simulink model "latest_coil"  (R2021b)
settings: Solver=FixedStepAuto  StartTime=-8e-3  StopTime=8e-3  FixedStep=1e-4  RelTol=1e-3
undefined symbols (not defined in the file or in its folder): X, Y, Z
libraries: sm_lib x15, nesl_utility x1
(part 2 of 2)

== matlab function latest_coil/Outer Coil/Coil 1/MATLAB Function3 ==
  data: X input; Hx_yp output; Y input; Z input; I input; Hy_yp output; Hz_yp output; Hx_yn output; Hy_yn output; Hz_yn output
function [Hx_yp, Hy_yp, Hz_yp, Hx_yn, Hy_yn, Hz_yn] = field_y(X, Y, Z, I)
n = 1;
gy = 520e-6;
% gx = 675e-6;
gz = 0;
m0 = 4*pi*1e-7;
k = 0.4e-3;
yp1 = -0.6e-3 - (n-1)*k;
yp2 = 0.6e-3 - (n-1)*k;
a_xp = gy;
a_zp = gz;
k_yp = 1./(4*pi*((a_xp-X).^2+(a_zp-Z).^2));
kyp = (yp2-Y)./((yp2-Y).^2+(a_xp-X).^2+(a_zp-Z).^2).^0.5;
k_2yp = (yp1-Y)./((yp1-Y).^2+(a_xp-X).^2+(a_zp-Z).^2).^0.5;

Hx_yp = -((a_zp-Z).*k_yp.*(kyp - k_2yp))*I*m0;
Hy_yp = zeros(size(X,1),size(Y,1),size(Z,1));
Hz_yp = (-(a_xp-X).*k_yp.*(kyp - k_2yp))*I*m0;

a_xn = -gy;
yn1 = -0.8e-3 - (n-1)*k;
yn2 = 0.8e-3 - (n-1)*k;
k_yn = 1./(4*pi*((a_xn-X).^2+(a_zp-Z).^2));
kyn = (yn2-Y)./((yn2-Y).^2+(a_xn-X).^2+(a_zp-Z).^2).^0.5;
k_2yn = (yn1-Y)./((yn1-Y).^2+(a_xn-X).^2+(a_zp-Z).^2).^0.5;

Hx_yn = ((a_zp-Z).*k_yn.*(kyn - k_2yn))*I*m0;
Hy_yn = zeros(size(X,1),size(Y,1),size(Z,1));
Hz_yn = ((a_xn-X).*k_yn.*(kyn - k_2yn))*I*m0;

end

== matlab function latest_coil/Outer Coil/Coil 1/MATLAB Function4 ==
  data: Hx_xp input; Hy_xp input; Hz_xp input; Hx output; Hx_xn input; Hy_xn input; Hy output; Hz output; Hz_xn input; Hx_yp input; Hy_yp input; Hz_yp input; Hx_yn input; Hy_yn input; Hz_yn input
function [Hx, Hy, Hz] = field_sum(Hx_xp, Hy_xp, Hz_xp, Hx_xn, Hy_xn, Hz_xn, Hx_yp, Hy_yp, Hz_yp, Hx_yn, Hy_yn, Hz_yn)
Hx = Hx_xp + Hx_xn + Hx_yp + Hx_yn;
Hy = Hy_xp + Hy_xn + Hy_yp + Hy_yn;
Hz = Hz_xp + Hz_xn + Hz_yp + Hz_yn;
end

== matlab function latest_coil/Outer Coil/Coil 2/MATLAB Function ==
  data: X input; Hx_xp output; Y input; Z input; I input; Hy_xp output; Hz_xp output; Hx_xn output; Hy_xn output; Hz_xn output
function [Hx_xp, Hy_xp, Hz_xp, Hx_xn, Hy_xn, Hz_xn] = field_x(X, Y, Z, I)
n = 1;
gx = 675e-6;
gz = 0;
m0 = 4*pi*1e-7;
k = 0.4e-3;
xp_1 = -0.8e-3 - (n-1)*k;
xp_2 = 0.8e-3 + (n-1)*k;
a_yp = gx; 
a_zp = gz;
k_p = 1./(4*pi*((a_yp-Y).^2+(a_zp-Z).^2));
kxp = (xp_2-X)./((xp_2-X).^2+(a_yp-Y).^2+(a_zp-Z).^2).^0.5;
k_2xp = (xp_1-X)./((xp_1-X).^2+(a_yp-Y).^2+(a_zp-Z).^2).^0.5;

Hx_xp = zeros(size(X,1),size(Y,1),size(Z,1));
Hy_xp = (-(a_zp-Z).*k_p.*(kxp - k_2xp))*I*m0;
Hz_xp = (-(a_yp-Y).*k_p.*(kxp - k_2xp))*I*m0;

a_yn = -gx;
xn_1 = -1e-3 - (n-1)*k;
xn_2 = 1e-3 + (n-1)*k;
k_n = 1./(4*pi*((a_yn-Y).^2+(a_zp-Z).^2));
kxn = (xn_2-X)./((xn_2-X).^2+(a_yn-Y).^2+(a_zp-Z).^2).^0.5;
k_2xn = (xn_1-X)./((xn_1-X).^2+(a_yn-Y).^2+(a_zp-Z).^2).^0.5;

Hx_xn = zeros(size(X,1),size(Y,1),size(Z,1));
Hy_xn = ((a_zp-Z).*k_n.*(kxn - k_2xn))*I*m0;
Hz_xn = ((a_yn-Y).*k_n.*(kxn - k_2xn))*I*m0;

end

== matlab function latest_coil/Outer Coil/Coil 2/MATLAB Function3 ==
  data: X input; Hx_yp output; Y input; Z input; I input; Hy_yp output; Hz_yp output; Hx_yn output; Hy_yn output; Hz_yn output
function [Hx_yp, Hy_yp, Hz_yp, Hx_yn, Hy_yn, Hz_yn] = field_y(X, Y, Z, I)
n = 1;
gy = 520e-6;
% gx = 675e-6;
gz = 0;
m0 = 4*pi*1e-7;
k = 0.4e-3;
yp1 = -0.6e-3 - (n-1)*k;
yp2 = 0.6e-3 - (n-1)*k;
a_xp = gy;
a_zp = gz;
k_yp = 1./(4*pi*((a_xp-X).^2+(a_zp-Z).^2));
kyp = (yp2-Y)./((yp2-Y).^2+(a_xp-X).^2+(a_zp-Z).^2).^0.5;
k_2yp = (yp1-Y)./((yp1-Y).^2+(a_xp-X).^2+(a_zp-Z).^2).^0.5;

Hx_yp = -((a_zp-Z).*k_yp.*(kyp - k_2yp))*I*m0;
Hy_yp = zeros(size(X,1),size(Y,1),size(Z,1));
Hz_yp = (-(a_xp-X).*k_yp.*(kyp - k_2yp))*I*m0;

a_xn = -gy;
yn1 = -0.8e-3 - (n-1)*k;
yn2 = 0.8e-3 - (n-1)*k;
k_yn = 1./(4*pi*((a_xn-X).^2+(a_zp-Z).^2));
kyn = (yn2-Y)./((yn2-Y).^2+(a_xn-X).^2+(a_zp-Z).^2).^0.5;
k_2yn = (yn1-Y)./((yn1-Y).^2+(a_xn-X).^2+(a_zp-Z).^2).^0.5;

Hx_yn = ((a_zp-Z).*k_yn.*(kyn - k_2yn))*I*m0;
Hy_yn = zeros(size(X,1),size(Y,1),size(Z,1));
Hz_yn = ((a_xn-X).*k_yn.*(kyn - k_2yn))*I*m0;

end

== matlab function latest_coil/Outer Coil/Coil 2/MATLAB Function4 ==
  data: Hx_xp input; Hy_xp input; Hz_xp input; Hx output; Hx_xn input; Hy_xn input; Hy output; Hz output; Hz_xn input; Hx_yp input; Hy_yp input; Hz_yp input; Hx_yn input; Hy_yn input; Hz_yn input
function [Hx, Hy, Hz] = field_sum(Hx_xp, Hy_xp, Hz_xp, Hx_xn, Hy_xn, Hz_xn, Hx_yp, Hy_yp, Hz_yp, Hx_yn, Hy_yn, Hz_yn)
Hx = Hx_xp + Hx_xn + Hx_yp + Hx_yn;
Hy = Hy_xp + Hy_xn + Hy_yp + Hy_yn;
Hz = Hz_xp + Hz_xn + Hz_yp + Hz_yn;
end

== matlab function latest_coil/Outer Coil/Coil 3/MATLAB Function ==
  data: X input; Hx_xp output; Y input; Z input; I input; Hy_xp output; Hz_xp output; Hx_xn output; Hy_xn output; Hz_xn output
function [Hx_xp, Hy_xp, Hz_xp, Hx_xn, Hy_xn, Hz_xn] = field_x(X, Y, Z, I)
n = 1;
gx = 675e-6;
gz = 0;
m0 = 4*pi*1e-7;
k = 0.4e-3;
xp_1 = -0.8e-3 - (n-1)*k;
xp_2 = 0.8e-3 + (n-1)*k;
a_yp = gx; 
a_zp = gz;
k_p = 1./(4*pi*((a_yp-Y).^2+(a_zp-Z).^2));
kxp = (xp_2-X)./((xp_2-X).^2+(a_yp-Y).^2+(a_zp-Z).^2).^0.5;
k_2xp = (xp_1-X)./((xp_1-X).^2+(a_yp-Y).^2+(a_zp-Z).^2).^0.5;

Hx_xp = zeros(size(X,1),size(Y,1),size(Z,1));
Hy_xp = (-(a_zp-Z).*k_p.*(kxp - k_2xp))*I*m0;
Hz_xp = (-(a_yp-Y).*k_p.*(kxp - k_2xp))*I*m0;

a_yn = -gx;
xn_1 = -1e-3 - (n-1)*k;
xn_2 = 1e-3 + (n-1)*k;
k_n = 1./(4*pi*((a_yn-Y).^2+(a_zp-Z).^2));
kxn = (xn_2-X)./((xn_2-X).^2+(a_yn-Y).^2+(a_zp-Z).^2).^0.5;
k_2xn = (xn_1-X)./((xn_1-X).^2+(a_yn-Y).^2+(a_zp-Z).^2).^0.5;

Hx_xn = zeros(size(X,1),size(Y,1),size(Z,1));
Hy_xn = ((a_zp-Z).*k_n.*(kxn - k_2xn))*I*m0;
Hz_xn = ((a_yn-Y).*k_n.*(kxn - k_2xn))*I*m0;

end

== matlab function latest_coil/Outer Coil/Coil 3/MATLAB Function3 ==
  data: X input; Hx_yp output; Y input; Z input; I input; Hy_yp output; Hz_yp output; Hx_yn output; Hy_yn output; Hz_yn output
function [Hx_yp, Hy_yp, Hz_yp, Hx_yn, Hy_yn, Hz_yn] = field_y(X, Y, Z, I)
n = 1;
gy = 520e-6;
% gx = 675e-6;
gz = 0;
m0 = 4*pi*1e-7;
k = 0.4e-3;
yp1 = -0.6e-3 - (n-1)*k;
yp2 = 0.6e-3 - (n-1)*k;
a_xp = gy;
a_zp = gz;
k_yp = 1./(4*pi*((a_xp-X).^2+(a_zp-Z).^2));
kyp = (yp2-Y)./((yp2-Y).^2+(a_xp-X).^2+(a_zp-Z).^2).^0.5;
k_2yp = (yp1-Y)./((yp1-Y).^2+(a_xp-X).^2+(a_zp-Z).^2).^0.5;

Hx_yp = -((a_zp-Z).*k_yp.*(kyp - k_2yp))*I*m0;
Hy_yp = zeros(size(X,1),size(Y,1),size(Z,1));
Hz_yp = (-(a_xp-X).*k_yp.*(kyp - k_2yp))*I*m0;

a_xn = -gy;
yn1 = -0.8e-3 - (n-1)*k;
yn2 = 0.8e-3 - (n-1)*k;
k_yn = 1./(4*pi*((a_xn-X).^2+(a_zp-Z).^2));
kyn = (yn2-Y)./((yn2-Y).^2+(a_xn-X).^2+(a_zp-Z).^2).^0.5;
k_2yn = (yn1-Y)./((yn1-Y).^2+(a_xn-X).^2+(a_zp-Z).^2).^0.5;

Hx_yn = ((a_zp-Z).*k_yn.*(kyn - k_2yn))*I*m0;
Hy_yn = zeros(size(X,1),size(Y,1),size(Z,1));
Hz_yn = ((a_xn-X).*k_yn.*(kyn - k_2yn))*I*m0;

end

== matlab function latest_coil/Outer Coil/Coil 3/MATLAB Function4 ==
  data: Hx_xp input; Hy_xp input; Hz_xp input; Hx output; Hx_xn input; Hy_xn input; Hy output; Hz output; Hz_xn input; Hx_yp input; Hy_yp input; Hz_yp input; Hx_yn input; Hy_yn input; Hz_yn input
function [Hx, Hy, Hz] = field_sum(Hx_xp, Hy_xp, Hz_xp, Hx_xn, Hy_xn, Hz_xn, Hx_yp, Hy_yp, Hz_yp, Hx_yn, Hy_yn, Hz_yn)
Hx = Hx_xp + Hx_xn + Hx_yp + Hx_yn;
Hy = Hy_xp + Hy_xn + Hy_yp + Hy_yn;
Hz = Hz_xp + Hz_xn + Hz_yp + Hz_yn;
end

== matlab function latest_coil/Outer Coil/Coil 4/MATLAB Function ==
  data: X input; Hx_xp output; Y input; Z input; I input; Hy_xp output; Hz_xp output; Hx_xn output; Hy_xn output; Hz_xn output
function [Hx_xp, Hy_xp, Hz_xp, Hx_xn, Hy_xn, Hz_xn] = field_x(X, Y, Z, I)
n = 1;
gx = 675e-6;
gz = 0;
m0 = 4*pi*1e-7;
k = 0.4e-3;
xp_1 = -0.8e-3 - (n-1)*k;
xp_2 = 0.8e-3 + (n-1)*k;
a_yp = gx; 
a_zp = gz;
k_p = 1./(4*pi*((a_yp-Y).^2+(a_zp-Z).^2));
kxp = (xp_2-X)./((xp_2-X).^2+(a_yp-Y).^2+(a_zp-Z).^2).^0.5;
k_2xp = (xp_1-X)./((xp_1-X).^2+(a_yp-Y).^2+(a_zp-Z).^2).^0.5;

Hx_xp = zeros(size(X,1),size(Y,1),size(Z,1));
Hy_xp = (-(a_zp-Z).*k_p.*(kxp - k_2xp))*I*m0;
Hz_xp = (-(a_yp-Y).*k_p.*(kxp - k_2xp))*I*m0;

a_yn = -gx;
xn_1 = -1e-3 - (n-1)*k;
xn_2 = 1e-3 + (n-1)*k;
k_n = 1./(4*pi*((a_yn-Y).^2+(a_zp-Z).^2));
kxn = (xn_2-X)./((xn_2-X).^2+(a_yn-Y).^2+(a_zp-Z).^2).^0.5;
k_2xn = (xn_1-X)./((xn_1-X).^2+(a_yn-Y).^2+(a_zp-Z).^2).^0.5;

Hx_xn = zeros(size(X,1),size(Y,1),size(Z,1));
Hy_xn = ((a_zp-Z).*k_n.*(kxn - k_2xn))*I*m0;
Hz_xn = ((a_yn-Y).*k_n.*(kxn - k_2xn))*I*m0;

end

== matlab function latest_coil/Inner Coil/Coil 1/MATLAB Function ==
  data: X input; Hx_xp output; Y input; Z input; I input; Hy_xp output; Hz_xp output; Hx_xn output; Hy_xn output; Hz_xn output; dBy_dy output; dBy_dz output
function [Hx_xp, Hy_xp, Hz_xp, Hx_xn, Hy_xn, Hz_xn, dBy_dy, dBy_dz] = field_x(X, Y, Z, I)
n = 1;
gx = 675e-6;
gz = 0;
m0 = 4*pi*1e-7;
k = 0.4e-3;
xp_1 = -0.8e-3 - (n-1)*k;
xp_2 = 0.8e-3 + (n-1)*k;
a_yp = gx; 
a_zp = gz;
k_p = 1./(4*pi*((a_yp-Y).^2+(a_zp-Z).^2));
kxp = (xp_2-X)./((xp_2-X).^2+(a_yp-Y).^2+(a_zp-Z).^2).^0.5;
k_2xp = (xp_1-X)./((xp_1-X).^2+(a_yp-Y).^2+(a_zp-Z).^2).^0.5;

Hx_xp = zeros(size(X,1),size(Y,1),size(Z,1));
Hy_xp = (-(a_zp-Z).*k_p.*(kxp - k_2xp))*I*m0;
Hz_xp = (-(a_yp-Y).*k_p.*(kxp - k_2xp))*I*m0;

a_yn = -gx;
xn_1 = -1e-3 - (n-1)*k;
xn_2 = 1e-3 + (n-1)*k;
k_n = 1./(4*pi*((a_yn-Y).^2+(a_zp-Z).^2));
kxn = (xn_2-X)./((xn_2-X).^2+(a_yn-Y).^2+(a_zp-Z).^2).^0.5;
k_2xn = (xn_1-X)./((xn_1-X).^2+(a_yn-Y).^2+(a_zp-Z).^2).^0.5;

Hx_xn = zeros(size(X,1),size(Y,1),size(Z,1));
Hy_xn = ((a_zp-Z).*k_n.*(kxn - k_2xn))*I*m0;
Hz_xn = ((a_yn-Y).*k_n.*(kxn - k_2xn))*I*m0;

k_1xp_3 = (xp_2-X)./((xp_2-X)^2+(a_yp-Y)^2+Z^2)^1.5;
k_2xp_3 = (xp_1-X)./((xp_1-X)^2+(a_yp-Y)^2+Z^2)^1.5;

k_1xn_3 = (xn_2-X)./((xn_2-X)^2+(a_yn-Y)^2+Z^2)^1.5;
k_2xn_3 = (xn_1-X)./((xn_1-X)^2+(a_yn-Y)^2+Z^2)^1.5;

hxp_x_1 = -(Z*k_p*(a_yp-Y))*I*m0;
hxp_x1_1 = (k_p*(kxp - k_2xp))*2*4*pi;
hxp_x2_1 = k_1xp_3 - k_2xp_3;
dByp_dy = hxp_x_1*(hxp_x1_1 + hxp_x2_1);

hxp_z_1 = (k_p)*I*m0;
hxp_z1_1 = (kxp - k_2xp)*(-1);
hxp_z2_1 = (k_p*(kxp - k_2xp)*(Z^2))*4*pi*2;
hxp_z3_1 = (k_1xp_3 - k_2xp_3)*(Z^2);
dByp_dz = hxp_z_1*(hxp_z1_1 + hxp_z2_1 + hxp_z3_1);

hxn_x_1 = -(Z*k_n*(a_yn-Y))*I*m0*(-1);
hxn_x1_1 = (k_n*(kxn - k_2xn))*2*4*pi;
hxn_x2_1 = k_1xn_3 - k_2xn_3;
dByn_dy = hxn_x_1*(hxn_x1_1 + hxn_x2_1);

hxn_z_1 = (k_n)*I*m0*(-1);
hxn_z1_1 = (kxn - k_2xn)*(-1);
hxn_z2_1 = (k_n*(kxn - k_2xn)*(Z^2))*4*pi*2;
hxn_z3_1 = (k_1xn_3 - k_2xn_3)*(Z^2);
dByn_dz = hxn_z_1*(hxn_z1_1 + hxn_z2_1 + hxn_z3_1);
dBy_dy = dByn_dy + dByp_dy;
dBy_dz = dByn_dz + dByp_dz;

end

== matlab function latest_coil/Outer Coil/Coil 4/MATLAB Function3 ==
  data: X input; Hx_yp output; Y input; Z input; I input; Hy_yp output; Hz_yp output; Hx_yn output; Hy_yn output; Hz_yn output
function [Hx_yp, Hy_yp, Hz_yp, Hx_yn, Hy_yn, Hz_yn] = field_y(X, Y, Z, I)
n = 1;
gy = 520e-6;
% gx = 675e-6;
gz = 0;
m0 = 4*pi*1e-7;
k = 0.4e-3;
yp1 = -0.6e-3 - (n-1)*k;
yp2 = 0.6e-3 - (n-1)*k;
a_xp = gy;
a_zp = gz;
k_yp = 1./(4*pi*((a_xp-X).^2+(a_zp-Z).^2));
kyp = (yp2-Y)./((yp2-Y).^2+(a_xp-X).^2+(a_zp-Z).^2).^0.5;
k_2yp = (yp1-Y)./((yp1-Y).^2+(a_xp-X).^2+(a_zp-Z).^2).^0.5;

Hx_yp = -((a_zp-Z).*k_yp.*(kyp - k_2yp))*I*m0;
Hy_yp = zeros(size(X,1),size(Y,1),size(Z,1));
Hz_yp = (-(a_xp-X).*k_yp.*(kyp - k_2yp))*I*m0;

a_xn = -gy;
yn1 = -0.8e-3 - (n-1)*k;
yn2 = 0.8e-3 - (n-1)*k;
k_yn = 1./(4*pi*((a_xn-X).^2+(a_zp-Z).^2));
kyn = (yn2-Y)./((yn2-Y).^2+(a_xn-X).^2+(a_zp-Z).^2).^0.5;
k_2yn = (yn1-Y)./((yn1-Y).^2+(a_xn-X).^2+(a_zp-Z).^2).^0.5;

Hx_yn = ((a_zp-Z).*k_yn.*(kyn - k_2yn))*I*m0;
Hy_yn = zeros(size(X,1),size(Y,1),size(Z,1));
Hz_yn = ((a_xn-X).*k_yn.*(kyn - k_2yn))*I*m0;

end

== matlab function latest_coil/Outer Coil/Coil 4/MATLAB Function4 ==
  data: Hx_xp input; Hy_xp input; Hz_xp input; Hx output; Hx_xn input; Hy_xn input; Hy output; Hz output; Hz_xn input; Hx_yp input; Hy_yp input; Hz_yp input; Hx_yn input; Hy_yn input; Hz_yn input
function [Hx, Hy, Hz] = field_sum(Hx_xp, Hy_xp, Hz_xp, Hx_xn, Hy_xn, Hz_xn, Hx_yp, Hy_yp, Hz_yp, Hx_yn, Hy_yn, Hz_yn)
Hx = Hx_xp + Hx_xn + Hx_yp + Hx_yn;
Hy = Hy_xp + Hy_xn + Hy_yp + Hy_yn;
Hz = Hz_xp + Hz_xn + Hz_yp + Hz_yn;
end

== matlab function latest_coil/Outer Coil/Coil 5/MATLAB Function ==
  data: X input; Hx_xp output; Y input; Z input; I input; Hy_xp output; Hz_xp output; Hx_xn output; Hy_xn output; Hz_xn output
function [Hx_xp, Hy_xp, Hz_xp, Hx_xn, Hy_xn, Hz_xn] = field_x(X, Y, Z, I)
n = 1;
gx = 675e-6;
gz = 0;
m0 = 4*pi*1e-7;
k = 0.4e-3;
xp_1 = -0.8e-3 - (n-1)*k;
xp_2 = 0.8e-3 + (n-1)*k;
a_yp = gx; 
a_zp = gz;
k_p = 1./(4*pi*((a_yp-Y).^2+(a_zp-Z).^2));
kxp = (xp_2-X)./((xp_2-X).^2+(a_yp-Y).^2+(a_zp-Z).^2).^0.5;
k_2xp = (xp_1-X)./((xp_1-X).^2+(a_yp-Y).^2+(a_zp-Z).^2).^0.5;

Hx_xp = zeros(size(X,1),size(Y,1),size(Z,1));
Hy_xp = (-(a_zp-Z).*k_p.*(kxp - k_2xp))*I*m0;
Hz_xp = (-(a_yp-Y).*k_p.*(kxp - k_2xp))*I*m0;

a_yn = -gx;
xn_1 = -1e-3 - (n-1)*k;
xn_2 = 1e-3 + (n-1)*k;
k_n = 1./(4*pi*((a_yn-Y).^2+(a_zp-Z).^2));
kxn = (xn_2-X)./((xn_2-X).^2+(a_yn-Y).^2+(a_zp-Z).^2).^0.5;
k_2xn = (xn_1-X)./((xn_1-X).^2+(a_yn-Y).^2+(a_zp-Z).^2).^0.5;

Hx_xn = zeros(size(X,1),size(Y,1),size(Z,1));
Hy_xn = ((a_zp-Z).*k_n.*(kxn - k_2xn))*I*m0;
Hz_xn = ((a_yn-Y).*k_n.*(kxn - k_2xn))*I*m0;

end

== matlab function latest_coil/Outer Coil/Coil 5/MATLAB Function3 ==
  data: X input; Hx_yp output; Y input; Z input; I input; Hy_yp output; Hz_yp output; Hx_yn output; Hy_yn output; Hz_yn output
function [Hx_yp, Hy_yp, Hz_yp, Hx_yn, Hy_yn, Hz_yn] = field_y(X, Y, Z, I)
n = 1;
gy = 520e-6;
% gx = 675e-6;
gz = 0;
m0 = 4*pi*1e-7;
k = 0.4e-3;
yp1 = -0.6e-3 - (n-1)*k;
yp2 = 0.6e-3 - (n-1)*k;
a_xp = gy;
a_zp = gz;
k_yp = 1./(4*pi*((a_xp-X).^2+(a_zp-Z).^2));
kyp = (yp2-Y)./((yp2-Y).^2+(a_xp-X).^2+(a_zp-Z).^2).^0.5;
k_2yp = (yp1-Y)./((yp1-Y).^2+(a_xp-X).^2+(a_zp-Z).^2).^0.5;

Hx_yp = -((a_zp-Z).*k_yp.*(kyp - k_2yp))*I*m0;
Hy_yp = zeros(size(X,1),size(Y,1),size(Z,1));
Hz_yp = (-(a_xp-X).*k_yp.*(kyp - k_2yp))*I*m0;

a_xn = -gy;
yn1 = -0.8e-3 - (n-1)*k;
yn2 = 0.8e-3 - (n-1)*k;
k_yn = 1./(4*pi*((a_xn-X).^2+(a_zp-Z).^2));
kyn = (yn2-Y)./((yn2-Y).^2+(a_xn-X).^2+(a_zp-Z).^2).^0.5;
k_2yn = (yn1-Y)./((yn1-Y).^2+(a_xn-X).^2+(a_zp-Z).^2).^0.5;

Hx_yn = ((a_zp-Z).*k_yn.*(kyn - k_2yn))*I*m0;
Hy_yn = zeros(size(X,1),size(Y,1),size(Z,1));
Hz_yn = ((a_xn-X).*k_yn.*(kyn - k_2yn))*I*m0;

end

== matlab function latest_coil/Outer Coil/Coil 5/MATLAB Function4 ==
  data: Hx_xp input; Hy_xp input; Hz_xp input; Hx output; Hx_xn input; Hy_xn input; Hy output; Hz output; Hz_xn input; Hx_yp input; Hy_yp input; Hz_yp input; Hx_yn input; Hy_yn input; Hz_yn input
function [Hx, Hy, Hz] = field_sum(Hx_xp, Hy_xp, Hz_xp, Hx_xn, Hy_xn, Hz_xn, Hx_yp, Hy_yp, Hz_yp, Hx_yn, Hy_yn, Hz_yn)
Hx = Hx_xp + Hx_xn + Hx_yp + Hx_yn;
Hy = Hy_xp + Hy_xn + Hy_yp + Hy_yn;
Hz = Hz_xp + Hz_xn + Hz_yp + Hz_yn;
end

== matlab function latest_coil/Gradinet ==
  data: df_xx output; Hx input; Hy input; Hz input; df_xy output; df_xz output; df_yx output; df_yy output; df_yz output; df_zx output; df_zy output; df_zz output
function [df_xx,df_xy,df_xz, df_yx,df_yy,df_yz,df_zx,df_zy,df_zz] = grad(Hx, Hy, Hz)
    [df_xx,df_xy,df_xz] = gradient(Hx,1e-3); %[dBx/dx, dBx/dy, dBx/dz]
    [df_yx,df_yy,df_yz] = gradient(Hy,1e-3); %[dBy/dx, dBy/dy, dBy/dz]
    [df_zx,df_zy,df_zz] = gradient(Hz,1e-3); %[dBz/dx, dBz/dy, dBz/dz]
end

== matlab function latest_coil/Force ==
  data: Fx output; df_xx input; df_xy input; df_xz input; Fy output; Fz output; df_yx input; df_yy input; df_yz input; df_zx input; df_zy input; df_zz input; Magentization input
function [Fx, Fy, Fz] = force(df_xx,df_xy,df_xz, df_yx,df_yy,df_yz,df_zx,df_zy,df_zz, Magentization)
    radius = 2e-3;
    height = 1e-3;
    vol_cy = pi*radius^2*height;
    F_xx = 0.1*Magentization*vol_cy * (df_xx)/m0 ;
    F_xy = 0.1*Magentization*vol_cy * (df_xy)/m0 ;
    F_xz = Magentization*vol_cy * (df_xz)/m0 ;
    F_yx = 0.1*Magentization*vol_cy * (df_yx)/m0 ;
    F_yy = 0.1*Magentization*vol_cy * (df_yy)/m0 ;
    F_yz = Magentization*vol_cy * (df_yz)/m0 ;
    F_zx = 0.1*Magentization*vol_cy * (df_zx)/m0 ;
    F_zy = 0.1*Magentization*vol_cy * (df_zy)/m0 ;
    F_zz = 0.1*Magentization*vol_cy * (df_zz)/m0 ;
    Fx = F_xx + F_xy + F_xz;
    Fy = F_yx + F_yy + F_yz;
    Fz = F_zx + F_zy + F_zz;
end

== matlab function latest_coil/MATLAB Function2 ==
  data: Ff_x output; Fext_x input; vx input
function Ff_x = friction(Fext_x,vx)
Coeff_of_Fric = 0.432;
g = 9.8;
mass_of_bot = 9.17345e-05;

% if  Fext_x < 0 && vx >= 0 %When force is in negative direction and velocity is in positive direction (impossible case) (Removing this case implies object doesn't move)
%     Ff_x = 0;
% elseif  Fext_x > 0 && vx <= 0 %When force is in positivedirection and velocity is in positive direction (impossible case)
%     Ff_x = 0;
% elseif  vx < 0 %When velocity is in negative direction friction is positive (Object is moving)
%     Ff_x = Coeff_of_Fric*mass_of_bot*g;
% elseif  vx > 0 %When velocity is in positive direction friction is negative (Object is moving)
%     Ff_x = -Coeff_of_Fric*mass_of_bot*g;
% elseif (abs(Fext_x) >= Coeff_of_Fric*mass_of_bot*g  &&  vx < 0 ) || (abs(Fext_x) >= Coeff_of_Fric*mass_of_bot*g && vx > 0) %When applied force greater than couloumb friction and 
%                                                                                                                        % moves is positive or negative direction, then Couloumb friction opposes that motion
%     Ff_x = -Coeff_of_Fric*mass_of_bot*g*sign(Fext_x);
% 
% elseif (abs(Fext_x) < Coeff_of_Fric*mass_of_bot*g && Fext_x~= 0) %When applied force less than Coloumb Friction but not equal to zero, Friction force is applied force
%     Ff_x = -Fext_x;
% else %When applied force is zero or when object not moving
%     Ff_x = -Fext_x;
% end

if abs(vx)<0.01
    if abs(Fext_x)>Coeff_of_Fric*mass_of_bot*g
        Ff_x=-Coeff_of_Fric*mass_of_bot*g*sign(Fext_x);
    else
        Ff_x=-Fext_x-vx;
    end
else
    Ff_x=-Coeff_of_Fric*mass_of_bot*g*sign(vx);
end

== matlab function latest_coil/Inner Coil/Coil 1/MATLAB Function4 ==
  data: Hx_xp input; Hy_xp input; Hz_xp input; Hx output; Hx_xn input; Hy_xn input; Hy output; Hz output; Hz_xn input; Hx_yp input; Hy_yp input; Hz_yp input; Hx_yn input; Hy_yn input; Hz_yn input
function [Hx, Hy, Hz] = field_sum(Hx_xp, Hy_xp, Hz_xp, Hx_xn, Hy_xn, Hz_xn, Hx_yp, Hy_yp, Hz_yp, Hx_yn, Hy_yn, Hz_yn)
Hx = Hx_xp + Hx_xn + Hx_yp + Hx_yn;
Hy = Hy_xp + Hy_xn + Hy_yp + Hy_yn;
Hz = Hz_xp + Hz_xn + Hz_yp + Hz_yn;
end

== matlab function latest_coil/Inner Coil/Coil 2/MATLAB Function ==
  data: X input; Hx_xp output; Y input; Z input; I input; Hy_xp output; Hz_xp output; Hx_xn output; Hy_xn output; Hz_xn output
function [Hx_xp, Hy_xp, Hz_xp, Hx_xn, Hy_xn, Hz_xn] = field_x(X, Y, Z, I)
n = 1;
gx = 675e-6;
gz = 0;
m0 = 4*pi*1e-7;
k = 0.4e-3;
xp_1 = -0.8e-3 - (n-1)*k;
xp_2 = 0.8e-3 + (n-1)*k;
a_yp = gx; 
a_zp = gz;
k_p = 1./(4*pi*((a_yp-Y).^2+(a_zp-Z).^2));
kxp = (xp_2-X)./((xp_2-X).^2+(a_yp-Y).^2+(a_zp-Z).^2).^0.5;
k_2xp = (xp_1-X)./((xp_1-X).^2+(a_yp-Y).^2+(a_zp-Z).^2).^0.5;

Hx_xp = zeros(size(X,1),size(Y,1),size(Z,1));
Hy_xp = (-(a_zp-Z).*k_p.*(kxp - k_2xp))*I*m0;
Hz_xp = (-(a_yp-Y).*k_p.*(kxp - k_2xp))*I*m0;

a_yn = -gx;
xn_1 = -1e-3 - (n-1)*k;
xn_2 = 1e-3 + (n-1)*k;
k_n = 1./(4*pi*((a_yn-Y).^2+(a_zp-Z).^2));
kxn = (xn_2-X)./((xn_2-X).^2+(a_yn-Y).^2+(a_zp-Z).^2).^0.5;
k_2xn = (xn_1-X)./((xn_1-X).^2+(a_yn-Y).^2+(a_zp-Z).^2).^0.5;

Hx_xn = zeros(size(X,1),size(Y,1),size(Z,1));
Hy_xn = ((a_zp-Z).*k_n.*(kxn - k_2xn))*I*m0;
Hz_xn = ((a_yn-Y).*k_n.*(kxn - k_2xn))*I*m0;

end
